simulink model "holder"  (R2015a)
settings: Solver=ode3  StartTime=0.0  StopTime=10.0  RelTol=1e-3
settings Model: Creator=thaodang  LastModifiedBy=thaodang

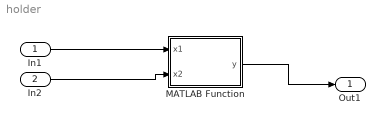
== system holder ==
  In1 : Inport  OutDataTypeStr=double
  In2 : Inport  Port=2  OutDataTypeStr=double
  MATLAB Function : MATLAB Function  TreatAsAtomicUnit=on
  Out1 : Outport
  wires:
  In1/1 -> MATLAB Function/1(x1)
  In2/1 -> MATLAB Function/2(x2)
  MATLAB Function/1(y) -> Out1/1

== matlab function holder/MATLAB Function ==
  data: x1 input; y output; x2 input
function y = fcn(x1, x2)
%#codegen


y = -(x2 + 47) * sin(sqrt(abs(x2 + x1 / 2.0 + 47))) - x1 * sin(sqrt(abs(x1 - (x2 + 47))));
